simulink model "DVBS2BentPipeLinkModel"  (R2021b)
settings: Solver=VariableStepAuto  StartTime=0.0  StopTime=0.025  RelTol=1e-3
PreLoadFcn:
  | modulationAndCodingMode = 'QPSK 1/4';
  | seed = 25;
  | ldpcFrameLength = 'Normal';
  | selDPD = false;
  | ulFreq = 4;  % GHz
  | selLvlBO = 1;  % '30 dB  (negligible nonlinearity)'
  | gsTxAntDiam = 4;  % m
  | selDoppler = 1;  %'0 Hz'
  | filterSpanInSymbols = 6;
  | sampPerSym = 8;
  | altitude = 35600;  % km
  | satRxAntDiam = 0.3;  % m
  | satRxNoiseFigure = 6;  % dB
  | chebyFilterOrder = 4;
  | satHPABackoff = 8;  % dB
  | dlFreq = 4.2;  % GHz
  | satTxAntDiam = 0.3;  % m
  | gsRxAntDiam = 1;  % m
  | gsRxNoiseFigure = 3;  % dB
  | selPhNo = 1;  % 'Negligible (-100 dBc/Hz @ 100 Hz)'
  | iqAmpImbal = 0;  % dB
  | iqPhImbal = 0;  % deg
  | dcOffsetPct = 0;  % percent of mean in-phase voltage
  | selDcOffset = false;
  | selCorrIQ = false;
  | selCorrDoppler = false;
  | LDPCNumIterations = 50;
  | DVBS2BentPipeInit(modulationAndCodingMode, seed, ...
  |   ldpcFrameLength, selDPD, ...
  |   ulFreq, selLvlBO, gsTxAntDiam, selDoppler, ...
  |   filterSpanInSymbols, sampPerSym, ...
  |   altitude, satRxAntDiam, satRxNoiseFigure, ...
  |   chebyFilterOrder, satHPABackoff, dlFreq, satTxAntDiam, ...
  |   gsRxAntDiam, gsRxNoiseFigure, selPhNo, ...
  |   iqAmpImbal, iqPhImbal, dcOffsetPct, ...
  |   selDcOffset, selCorrIQ, selCorrDoppler, ...
  |   LDPCNumIterations);
  | 
  | clear modulationAndCodingMode seed ldpcFrameLength selDPD
  | clear ulFreq selLvlBO gsTxAntDiam selDoppler
  | clear filterSpanInSymbols sampPerSym
  | clear altitude satRxAntDiam satRxNoiseFigure
  | clear chebyFilterOrder satHPABackoff dlFreq satTxAntDiam
  | clear gsRxAntDiam gsRxNoiseFigure selPhNo
  | clear iqAmpImbal iqPhImbal dcOffsetPct
  | clear selDcOffset selCorrIQ selCorrDoppler
  | clear LDPCNumIterations
undefined symbols (not defined in the file or in its folder): paramRFSatLink
libraries: dspstat3 x17, commrflib2 x9, commrfcorlib x5, commblkcod2 x4, dspsigops x4, commsink2 x3, commutil2 x3, dspmathops x3, commblkintrlv2 x2, dspobslib x2, commdigbbndpm3 x2, commfilt2 x2
(part 1 of 2)
settings Model: Creator=The MathWorks, Inc.  LastModifiedBy=lenovo

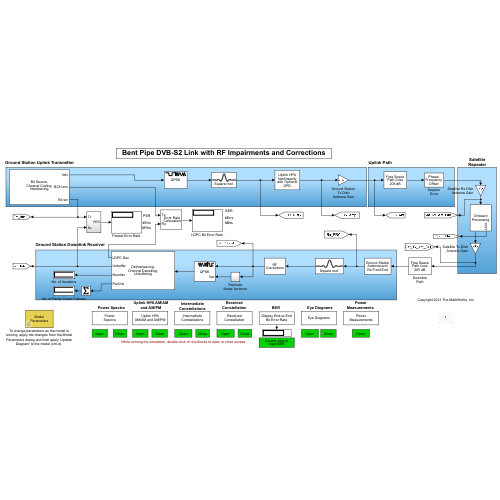
[thumbnail: Simulink's stored preview of the top-level diagram]
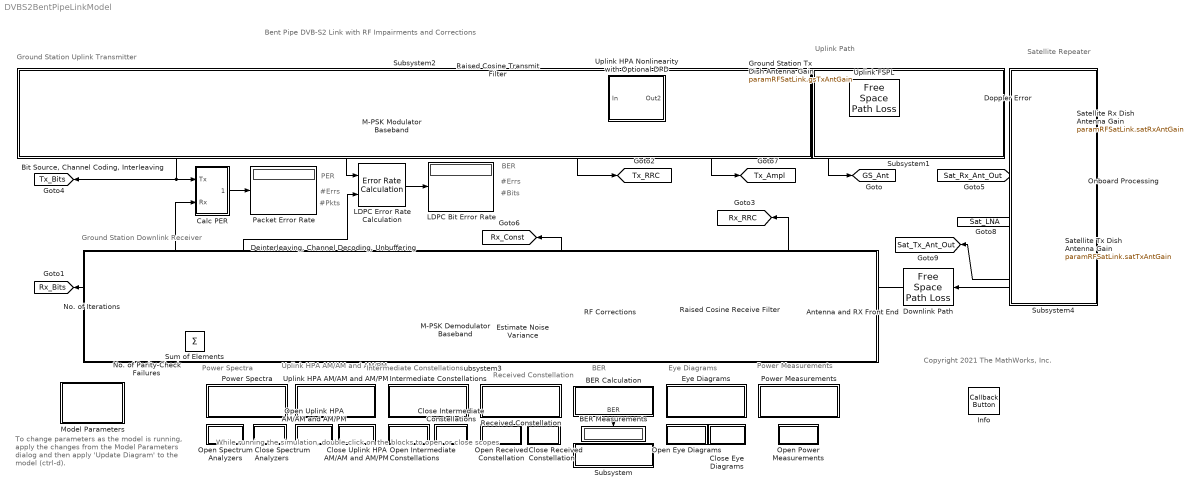
== system DVBS2BentPipeLinkModel ==
  note: Copyright 2021 The MathWorks, Inc.
  note: BER
  note: PER
  note: Satellite
      | Repeater
  note: Ground Station Uplink Transmitter
  note: To change parameters as the model is running, apply the changes from the Model Parameters dialog and then apply 'Update Diagram' to the model (ctrl-d).
  note: Received
      | Constellation
  note: Eye Diagrams
  note: BER
  note: While running the simulation, double-click on the blocks to open or close scopes
  note: Uplink HPA AM/AM
      | and AM/PM
  note: #Pkts
  note: #Errs
  note: Ground Station Downlink Receiver
  note: Bent Pipe DVB-S2 Link with RF Impairments and Corrections
  note: #Bits
  note: #Errs
  note: Power Spectra
  note: Intermediate
      | Constellations
  note: Uplink Path
  note: Power
      | Measurements
  Antenna and RX Front End : Subsystem
      mask Display: disp('Ground Station\nAntenna and\nRx Front End')
  BER Calculation : Subsystem
      mask Display: disp('Display End-to-End\nBit Error Rate');
  BER Measurements : Display
      settings: Format=short_e
  "Bit Source, Channel Coding, Interleaving" : Subsystem
      mask Display:
      | disp('Bit Source,\nChannel Coding,\nInterleaving\n')
      | port_label('output',1,'Intlv')
      | port_label('output',2,'BCH enc')
      | port_label('output',3,'Bit src')
  Calc PER : Subsystem
  Close Intermediate Constellations : Subsystem
      settings: OpenFcn=|
      | % RRC signal before and after uplink HPA
      | ULHPACD = [bdroot '/Intermediate Constellations/RRC Signal Before and After Uplink HPA'];
      | close_system(ULHPACD);
      | % set_param(ULHPACD,'OpenScopeAtSimStart','off');
      | clear ULHPACD
      | 
      | % Constellations onboard satellite
      | onboardCD = [bdroot '/Intermediate Constellations/Onboard Constellations'];
      | close_system(onboardCD);
      | % set_param(onboardCD,'OpenScopeAtSimStart','off');
      | clear onboardCD
      mask Display: disp('Close');
  Close Eye Diagrams : Subsystem
      settings: OpenFcn=|
      | % Satellite AGC Output Eye Diagram
      | satAGCED = [bdroot '/Eye Diagrams/Sat AGC Output Eye Diagram'];
      | close_system(satAGCED);
      | % set_param(satAGCED,'OpenScopeAtSimStart','off');
      | clear satAGCED
      | 
      | % Chebyshev Filter Output Eye Diagram
      | chebyFiltED = [bdroot '/Eye Diagrams/Chebyshev Filter Output Eye Diagram'];
      | close_system(chebyFiltED);
      | % set_param(chebyFiltED,'OpenScopeAtSimStart','off');
      | clear chebyFiltED
      | 
      | % Rx Eye Diagram
      | rxED = [bdroot '/Eye Diagrams/Rx Eye Diagram'];
      | close_system(rxED);
      | % set_param(rxED,'OpenScopeAtSimStart','off');
      | clear rxED
      mask Display: disp('Close');
  Close Received Constellation : Subsystem
      settings: OpenFcn=|
      | rxCD = [bdroot '/Received Constellation/Received Constellation'];
      | close_system(rxCD);
      | % set_param(rxCD,'OpenScopeAtSimStart','off');
      | clear rxCD
      mask Display: disp('Close');
  Close Spectrum Analyzers : Subsystem
      settings: OpenFcn=|
      | % Tx and rx spectra
      | txrxSA = [bdroot '/Power Spectra/Ground Station Tx and Rx Spectra'];
      | close_system(txrxSA);
      | % set_param(txrxSA,'OpenScopeAtSimStart','off');
      | clear txrxSA
      | 
      | % Spectra onboard satellite
      | satSA = [bdroot '/Power Spectra/Onboard Spectra'];
      | close_system(satSA);
      | % set_param(satSA,'OpenScopeAtSimStart','off');
      | clear satSA
      mask Display: disp('Close');
  Close Uplink HPA AM/AM and AM/PM : Subsystem
      settings: OpenFcn=|
      | % AM/AM
      | AMAMplot = [bdroot '/Uplink HPA AM//AM and AM//PM/Input&Output of HPA/HPA AM to AM'];
      | close_system(AMAMplot);
      | % set_param(AMAMplot,'OpenScopeAtSimStart','off');
      | clear AMAMplot
      | 
      | % AM/PM
      | AMPMplot = [bdroot '/Uplink HPA AM//AM and AM//PM/Input&Output of HPA/HPA AM to PM'];
      | close_system(AMPMplot);
      | % set_param(AMPMplot,'OpenScopeAtSimStart','off');
      | clear AMPMplot
      mask Display: disp('Close');
  "Deinterleaving, Channel Decoding, Unbuffering" : Subsystem
      mask Display:
      | disp('Deinterleaving,\nChannel Decoding,\nUnbuffering')
      | port_label('output',1,'LDPC Dec')
      | port_label('output',2,'Unbuffer')
      | port_label('output',3,'NumIter')
      | port_label('output',4,'ParChk')
  Doppler Error : commrflib2/Phase// Frequency Offset  phaseOffset=0  freqPort=off  freqOffset=paramRFSatLink.DoppOffset
  Downlink Path : commrflib2/Free Space Path Loss  mode=Distance and Frequency  dB=180  d=paramRFSatLink.Altitude  fc="paramRFSatLink.DownlinkFrequency * 1e3  % GHz to MHz"
      settings: SourceProductBaseCode=CM
  Estimate Noise Variance : Subsystem
  Eye Diagrams : Subsystem
      mask Display: disp('Eye Diagrams');
  Ground Station Tx Dish Antenna Gain : Gain  Gain=paramRFSatLink.gsTxAntGain  SaturateOnIntegerOverflow=on  OutDataTypeStr=Inherit: Same as input  ParamDataTypeStr=Inherit: Same as input
  Info : CallbackButton  ButtonText=?
      settings: ClickFcn=showExample('satcom/DVBS2BentPipeSimulationWithRFImpairmentsAndCorrectionsExample')
  Intermediate Constellations : Subsystem
      mask Display: disp('Intermediate\nConstellations')
  LDPC Bit Error Rate : Display
  LDPC Error Rate Calculation : commsink2/Error Rate Calculation  N=paramRFSatLink.LDPCLinkRecDelay  st_delay=paramRFSatLink.BCHCodewordLength  cp_mode=Entire frame  subframe=[]  PMode=Port  WsName=ErrorVec  RsMode2=off  stop=off  numErr=100  maxBits=1e6
  M-PSK Demodulator Baseband : commdigbbndpm3/M-PSK Demodulator Baseband  M=paramRFSatLink.ModulationOrder  OutType=Bit  DecType=Approximate log-likelihood ratio  VarSource=Port  Variance=1/(1+10^(paramRFSatLink.EsNodB/10))  Dec=User-defined  Mapping=paramRFSatLink.SymbolMapping  Ph=paramRFSatLink.PhaseOffset  outDtype1=double  outDtype2=double  derotateFactorWordLen=16  derotateFactorDataTypeStr=Inherit: Same word length as input  derotateFactorLastDataTypeStr=Inherit: Same word length as input
  M-PSK Modulator Baseband : commdigbbndpm3/M-PSK Modulator Baseband  M=paramRFSatLink.ModulationOrder  InType=Bit  Enc=User-defined  Mapping=paramRFSatLink.SymbolMapping  Ph=paramRFSatLink.PhaseOffset  outDtype=double  outWordLen=16  outUDDataType=sfix(16)  outFracLenMode=Best precision  outFracLen=15  outDataTypeStr=double  outLastDataTypeStr=double
  Model Parameters : Subsystem  mask(Model Parameters){modulationAndCodingMode=QPSK 1/4, seed=23, ldpcFrameLength=Normal, selDPD=off, ulFreq=14, selLvlBO=30 dB  (negligible nonlinearity), gsTxAntDiam=8, dopplerFreq=0, filterSpanInSymbols=6, sampPerSym=8, altitude=35600, satRxAntDiam=2, satRxNoiseFigure=6, chebyFilterOrder=4, satHPABackoff=4, dlFreq=12, satTxAntDiam=2, gsRxAntDiam=8, gsRxNoiseFigure=3, selPhNo=Negligible (-100 dBc/Hz @ 100 Hz), iqAmpImbal=0, iqPhImbal=0, dcOffsetPct=0, selCorrDCOffset=off, selCorrIQ=off, selCorrDoppler=off, LDPCNumIterations=50}
      mask prompts: modulationAndCodingMode "Mode:"; seed "Seed (for random data and noise):"; ldpcFrameLength "LDPC frame length:"; selDPD "Digital predistortion"; ulFreq "Uplink frequency (GHz):"; selLvlBO "HPA backoff level:"; gsTxAntDiam "Transmit antenna diameter (m):"; dopplerFreq "Doppler error (Hz):"; filterSpanInSymbols "Filter span (symbols):"; sampPerSym "Filter output samples per symbol:"; altitude "Satellite altitude (km):"; satRxAntDiam "Receive antenna diameter (m):"; satRxNoiseFigure "Receiver noise figure (dB):"; chebyFilterOrder "Chebyshev filter order:"; satHPABackoff "HPA backoff level (dB):"; dlFreq "Downlink frequency (GHz):"; satTxAntDiam "Transmit antenna diameter (m):"; gsRxAntDiam "Receive antenna diameter (m):"; gsRxNoiseFigure "Receiver noise figure (dB):"; selPhNo "Phase noise:"; iqAmpImbal "I/Q amplitude imbalance (dB):"; iqPhImbal "I/Q phase imbalance (deg):"; dcOffsetPct "In-phase DC offset (%):"; selCorrDCOffset "DC offset correction"; selCorrIQ "I/Q imbalance correction"; selCorrDoppler "Doppler correction"; LDPCNumIterations "Number of LDPC decoder iterations:"
      mask help:
      | Select the scenarios from the mask to change the link parameters. Each of the mask parameters sets the parameters in the corresponding RF impairment or corresponding correction block(s).
      |
      | To make changes as the model is running, apply the changes from this dialog and then apply Update Diagram to the model (crtl-d).
      mask init:
      | DVBS2BentPipeInit(modulationAndCodingMode, seed, ...
      |   ldpcFrameLength, selDPD, ulFreq, selLvlBO, ...
      |   gsTxAntDiam, dopplerFreq, filterSpanInSymbols, ...
      |   sampPerSym, altitude, satRxAntDiam, satRxNoiseFigure, ...
      |   chebyFilterOrder, satHPABackoff, dlFreq, satTxAntDiam, ...
      |   gsRxAntDiam, gsRxNoiseFigure, selPhNo, ...
      |   iqAmpImbal, iqPhImbal, dcOffsetPct, ...
      |   selCorrDCOffset, selCorrIQ, selCorrDoppler, ...
      |   LDPCNumIterations);
      mask Help: helpview(commdhelp);
      mask TypeOptions modulationAndCodingMode: QPSK 1/4 | QPSK 1/3 | QPSK 2/5 | QPSK 1/2 | QPSK 3/5 | QPSK 2/3 | QPSK 3/4 | QPSK 4/5 | QPSK 5/6 | QPSK 8/9 | QPSK 9/10 | 8PSK 3/5 | 8PSK 2/3 | 8PSK 3/4 | 8PSK 5/6 | 8PSK 8/9 | 8PSK 9/10
      mask TypeOptions ldpcFrameLength: Normal | Short
      mask TypeOptions selLvlBO: 30 dB  (negligible nonlinearity) | 7 dB  (moderate nonlinearity) | 1 dB  (severe nonlinearity)
      mask TypeOptions selPhNo: Negligible (-100 dBc/Hz @ 100 Hz) | Low  (-55 dBc/Hz @ 100 Hz) | High  (-48 dBc/Hz @ 100 Hz)
      mask DialogControl uplinkTab Prompt: Uplink
      mask DialogControl satelliteTab Prompt: Satellite
      mask DialogControl downlinkTab Prompt: Downlink
      mask Display: disp('Model\nParameters');
  No. of Iterations : Display
  No. of Parity-Check Failures : Display
  Onboard Processing : Subsystem
      mask Display:
      | disp('Onboard\nProcessing');
      | port_label('output',2,'LNA');
  Open Intermediate Constellations : Subsystem
      settings: OpenFcn=|
      | % RRC signal before and after uplink HPA
      | ULHPACD = [bdroot '/Intermediate Constellations/RRC Signal Before and After Uplink HPA'];
      | open_system(ULHPACD);
      | % set_param(ULHPACD,'OpenScopeAtSimStart','on');
      | clear ULHPACD
      | 
      | % Constellations onboard satellite
      | onboardCD = [bdroot '/Intermediate Constellations/Onboard Constellations'];
      | open_system(onboardCD);
      | % set_param(onboardCD,'OpenScopeAtSimStart','on');
      | clear onboardCD
      mask Display: disp('Open');
  Open Eye Diagrams : Subsystem
      settings: OpenFcn=|
      | % Satellite AGC Output Eye Diagram
      | satAGCED = [bdroot '/Eye Diagrams/Sat AGC Output Eye Diagram'];
      | open_system(satAGCED);
      | % set_param(satAGCED,'OpenScopeAtSimStart','on');
      | clear satAGCED
      | 
      | % Chebyshev Filter Output Eye Diagram
      | chebyFiltED = [bdroot '/Eye Diagrams/Chebyshev Filter Output Eye Diagram'];
      | open_system(chebyFiltED);
      | % set_param(chebyFiltED,'OpenScopeAtSimStart','on');
      | clear chebyFiltED
      | 
      | % Rx Eye Diagram
      | rxED = [bdroot '/Eye Diagrams/Rx Eye Diagram'];
      | open_system(rxED);
      | % set_param(rxED,'OpenScopeAtSimStart','on');
      | clear rxED
      mask Display: disp('Open');
  Open Power Measurements : Subsystem
      settings: OpenFcn=open_system([bdroot '/Power Measurements']);
      mask Display: disp('Open');
  Open Received Constellation : Subsystem
      settings: OpenFcn=|
      | rxCD = [bdroot '/Received Constellation/Received Constellation'];
      | open_system(rxCD);
      | % set_param(rxCD,'OpenScopeAtSimStart','on');
      | clear rxCD
      mask Display: disp('Open');
  Open Spectrum Analyzers : Subsystem
      settings: OpenFcn=|
      | % Tx and rx spectra
      | txrxSA = [bdroot '/Power Spectra/Ground Station Tx and Rx Spectra'];
      | open_system(txrxSA);
      | % set_param(txrxSA,'OpenScopeAtSimStart','on');
      | clear txrxSA
      | 
      | % Spectra onboard satellite
      | satSA = [bdroot '/Power Spectra/Onboard Spectra'];
      | open_system(satSA);
      | % set_param(satSA,'OpenScopeAtSimStart','on');
      | clear satSA
      mask Display: disp('Open');
  Open Uplink HPA AM/AM and AM/PM : Subsystem
      settings: OpenFcn=|
      | % AM/AM
      | AMAMplot = [bdroot '/Uplink HPA AM//AM and AM//PM/Input&Output of HPA/HPA AM to AM'];
      | open_system(AMAMplot);
      | % set_param(AMAMplot,'OpenScopeAtSimStart','on');
      | clear AMAMplot
      | 
      | % AM/PM
      | AMPMplot = [bdroot '/Uplink HPA AM//AM and AM//PM/Input&Output of HPA/HPA AM to PM'];
      | open_system(AMPMplot);
      | % set_param(AMPMplot,'OpenScopeAtSimStart','on');
      | clear AMPMplot
      mask Display: disp('Open');
  Packet Error Rate : Display
  Power Measurements : Subsystem
      mask Display: disp('Power\nMeasurements')
  Power Spectra : Subsystem
      mask Display: disp('Power\nSpectra')
  RF Corrections : Subsystem
      mask Display: disp('RF\nCorrections')
  Raised Cosine Receive Filter : commfilt2/Raised Cosine Receive Filter  filtType=Square root  R=0.25  filtSpan=paramRFSatLink.FilterSpanInSymbols  N=paramRFSatLink.SamplesPerSymbol  downFactor=paramRFSatLink.SamplesPerSymbol  downOffset=0  filterGain=1/sqrt(paramRFSatLink.SamplesPerSymbol)  InputProcessing=Columns as channels (frame based)  RateOptions=Enforce single-rate processing  framing=Mute  checkCoeff=off  variableName=rcRxFilt  currentFiltSpan=paramRFSatLink.FilterSpan  D=(paramRFSatLink.FilterSpan)/2  inputOffset=0  sampMode=Mute  saveAsFlag=0  rateMode=Downsampling  checkGain=Normalized  launchFVT=off  roundingMode=Floor  overflowMode=off  coeffDataTypeStr=Inherit: Same word length as input  coeffMin=[]  coeffMax=[]  coeffLastDataTypeStr=Inherit: Same word length as input  accumDataTypeStr=Inherit: Same as product output  accumLastDataTypeStr=Inherit: Same as product output  outputDataTypeStr=Inherit: Same as accumulator  outputMin=[]  outputMax=[]  outputLastDataTypeStr=Inherit: Same as accumulator
  Raised Cosine Transmit Filter : commfilt2/Raised Cosine Transmit Filter  filtType=Square root  R=0.25  filtSpan=paramRFSatLink.FilterSpanInSymbols  N=paramRFSatLink.SamplesPerSymbol  filterGain=sqrt(paramRFSatLink.SamplesPerSymbol)  InputProcessing=Columns as channels (frame based)  RateOptions=Enforce single-rate processing  framing=Mute  checkCoeff=off  variableName=rcTxFilt  checkGain=Normalized  sampMode=Mute  saveAsFlag=0  currentFiltSpan=paramRFSatLink.FilterSpan  D=(paramRFSatLink.FilterSpan)/2  launchFVT=off  roundingMode=Floor  overflowMode=off  coeffDataTypeStr=Inherit: Same word length as input  coeffMin=[]  coeffMax=[]  coeffLastDataTypeStr=Inherit: Same word length as input  outputDataTypeStr=Inherit: Same as accumulator  outputMin=[]  outputMax=[]  outputLastDataTypeStr=Inherit: Same as accumulator
  Received Constellation : Subsystem
      mask Display: disp('Received\nConstellation')
  Satellite Rx Dish Antenna Gain : Gain  Gain=paramRFSatLink.satRxAntGain  SaturateOnIntegerOverflow=on  OutDataTypeStr=Inherit: Same as input  ParamDataTypeStr=Inherit: Same as input
  Satellite Tx Dish Antenna Gain : Gain  Gain=paramRFSatLink.satTxAntGain  SaturateOnIntegerOverflow=on  OutDataTypeStr=Inherit: Same as input  ParamDataTypeStr=Inherit: Same as input
  Subsystem : Subsystem
      settings: OpenFcn=|
      | % Set value to reset BER
      | warning('off', 'Simulink:Engine:NonTunableVarChanged');
      | paramRFSatLink.resetBER = 1;
      | set_param(bdroot, 'SimulationCommand', 'update');
      | pause(0.1)
      | 
      | % Set value so that BER is not continually reset
      | paramRFSatLink.resetBER = 0;
      | set_param(bdroot, 'SimulationCommand', 'update');
      | warning('on', 'Simulink:Engine:NonTunableVarChanged');
      mask Display: disp('Double-click to\nreset BER')
  Subsystem1 : Subsystem
  Subsystem2 : Subsystem
  Subsystem3 : Subsystem
  Subsystem4 : Subsystem
  Sum of Elements : Sum  Inputs=+
  Uplink FSPL : commrflib2/Free Space Path Loss  mode=Distance and Frequency  dB=180  d=paramRFSatLink.Altitude  fc="paramRFSatLink.UplinkFrequency * 1e3  % GHz to MHz"
      settings: SourceProductBaseCode=CM
  Uplink HPA Nonlinearity with Optional DPD : Subsystem
      mask Display: disp('Uplink HPA\nNonlinearity\nwith Optional\nDPD')
  Uplink HPA AM/AM and AM/PM : Subsystem
      mask Display: disp('Uplink HPA\nAM/AM and AM/PM')
  tag scope: GS_Ant=global, Rx_Bits=global, Rx_Const=global, Rx_RRC=global, Sat_LNA=global, Sat_Rx_Ant_Out=global, Sat_Tx_Ant_Out=global, Tx_Ampl=global, Tx_Bits=global, Tx_RRC=global
  wires:
  Satellite Rx Dish Antenna Gain/1 -> Onboard Processing/1(In1), [Sat_Rx_Ant_Out]
  LDPC Error Rate Calculation/1 -> LDPC Bit Error Rate/1
  Raised Cosine Transmit Filter/1 -> Uplink HPA Nonlinearity with Optional DPD/1(In), [Tx_RRC]
  Sum of Elements/1 -> No. of Parity-Check Failures/1
  Antenna and RX Front End/1(Out1) -> Raised Cosine Receive Filter/1, [Rx_RRC]
  Doppler Error/1 -> Satellite Rx Dish Antenna Gain/1
  BER Calculation/1(BER) -> BER Measurements/1
  Satellite Tx Dish Antenna Gain/1 -> [Sat_Tx_Ant_Out], Downlink Path/1
  Estimate Noise Variance/1(Out1) -> M-PSK Demodulator Baseband/2
  Calc PER/1(PER) -> Packet Error Rate/1
  Uplink HPA Nonlinearity with Optional DPD/1(Out2) -> Ground Station Tx Dish Antenna Gain/1, [Tx_Ampl]
  Downlink Path/1 -> Antenna and RX Front End/1(In1)
  Uplink FSPL/1 -> Doppler Error/1
  Ground Station Tx Dish Antenna Gain/1 -> [GS_Ant], Uplink FSPL/1
  "Bit Source, Channel Coding, Interleaving"/3(Bit Src) -> [Tx_Bits], Calc PER/1(Tx)
  "Bit Source, Channel Coding, Interleaving"/1(Intlv Out) -> M-PSK Modulator Baseband/1
  "Bit Source, Channel Coding, Interleaving"/2(BCH Enc Out) -> LDPC Error Rate Calculation/1
  "Deinterleaving, Channel Decoding, Unbuffering"/2(Unbuffer) -> [Rx_Bits], Calc PER/2(Rx)
  M-PSK Demodulator Baseband/1 -> "Deinterleaving, Channel Decoding, Unbuffering"/1(QPSK Demod)
  "Deinterleaving, Channel Decoding, Unbuffering"/1(LDPC Dec) -> LDPC Error Rate Calculation/2
  "Deinterleaving, Channel Decoding, Unbuffering"/3(NumIter) -> No. of Iterations/1
  "Deinterleaving, Channel Decoding, Unbuffering"/4(ParChk) -> Sum of Elements/1
  Onboard Processing/1(Out2) -> Satellite Tx Dish Antenna Gain/1
  Onboard Processing/2(LNA Out) -> [Sat_LNA]
  Raised Cosine Receive Filter/1 -> RF Corrections/1(In1)
  M-PSK Modulator Baseband/1 -> Raised Cosine Transmit Filter/1
  RF Corrections/1(Out1) -> Estimate Noise Variance/1(In1), M-PSK Demodulator Baseband/1, [Rx_Const]

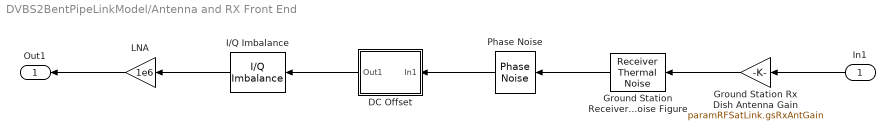
== system DVBS2BentPipeLinkModel/Antenna and RX Front End ==
  In1 : Inport
  DC Offset : Subsystem
      mask Display: disp('DC Offset')
  Ground Station Receiver Noise Figure : commrflib2/Receiver Thermal Noise  method=Noise figure  ntemp=paramRFSatLink.RXTemp  nfigure=paramRFSatLink.GSRxNoiseFigure  nfactor=2  add290KAntennaNoise=off  seed=67987
      settings: SourceProductBaseCode=CM
  Ground Station Rx Dish Antenna Gain : Gain  Gain=paramRFSatLink.gsRxAntGain  SaturateOnIntegerOverflow=on  OutDataTypeStr=Inherit: Same as input  ParamDataTypeStr=Inherit: Same as input
  I/Q Imbalance : commrflib2/I//Q Imbalance  ampImbal=paramRFSatLink.IQAmpImbal  phsImbal=paramRFSatLink.IQPhImbal  Idc=0  Qdc=0
      settings: SourceProductBaseCode=CM
  LNA : Gain  Gain=1e6
  Phase Noise : impairlib/Phase Noise  Level=paramRFSatLink.PhaseNoise  FrequencyOffset=100  SampleRate=2e5  RandomStream=mt19937ar with seed  Seed=2137  SimulateUsing=Interpreted execution
      settings: SourceProductBaseCode=CM,AM,SX
  Out1 : Outport  VectorParamsAs1DForOutWhenUnconnected=off
  wires:
  LNA/1 -> Out1/1
  Ground Station Receiver Noise Figure/1 -> Phase Noise/1
  In1/1 -> Ground Station Rx Dish Antenna Gain/1
  I/Q Imbalance/1 -> LNA/1
  Ground Station Rx Dish Antenna Gain/1 -> Ground Station Receiver Noise Figure/1
  DC Offset/1(Out1) -> I/Q Imbalance/1
  Phase Noise/1 -> DC Offset/1(In1)

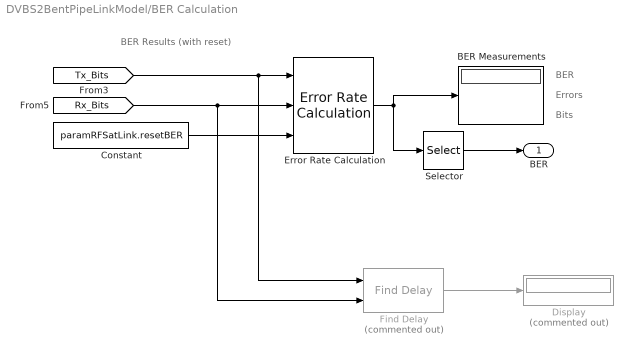
== system DVBS2BentPipeLinkModel/BER Calculation ==
  note: BER
  note: Errors
  note: Bits
  note: BER Results (with reset)
  BER Measurements : Display
  Constant : Constant  Value=paramRFSatLink.resetBER  SampleTime=Inf
  Display : Display  Commented=on
  Error Rate Calculation : commsink2/Error Rate Calculation  N=paramRFSatLink.FullLinkRecDelay  st_delay=paramRFSatLink.BCHMessageLength  cp_mode=Entire frame  subframe=[]  PMode=Port  WsName=ErrorVec  RsMode2=on  stop=off  numErr=200  maxBits=1e6
  Find Delay : commutil2/Find Delay  Commented=on  corrLength=15000  chgSigOP=off  stopUpdate=off  numConstDelay=3
      settings: SourceProductBaseCode=CM
  Selector : Selector  InputPortWidth=3  IndexOptions=Index vector (dialog)  Indices=[1]  OutputSizes=1
  BER : Outport  VectorParamsAs1DForOutWhenUnconnected=off
  wires:
  [Rx_Bits] -> Find Delay/2, Error Rate Calculation/2
  Error Rate Calculation/1 -> Selector/1, BER Measurements/1
  Constant/1 -> Error Rate Calculation/3
  Selector/1 -> BER/1
  [Tx_Bits] -> Find Delay/1, Error Rate Calculation/1
  Find Delay/1 -> Display/1

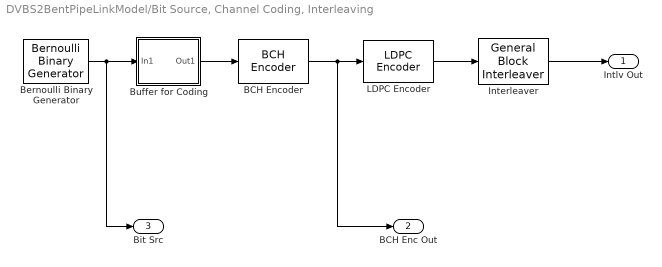
== system DVBS2BentPipeLinkModel/Bit Source, Channel Coding, Interleaving ==
  BCH Encoder : commblkcod2/BCH Encoder  n=paramRFSatLink.BCHCodewordLength  k=paramRFSatLink.BCHMessageLength  specShortening=off  shortenedK=5  specGenPoly=on  genPoly=paramRFSatLink.BCHGeneratorPoly  specPrimPoly=on  prPoly=paramRFSatLink.BCHPrimitivePoly  specDisableGenCheck=on  specPuncture=off  punctVec=[ones(8,1); zeros(2,1)]
      settings: SourceProductBaseCode=CM
  Bernoulli Binary Generator : commrandsrc3/Bernoulli Binary Generator  ProbabilityOfZero=0.5  SeedSource=Parameter  Seed=paramRFSatLink.Seed  SampleTime=paramRFSatLink.BitPeriod  SamplesPerFrame=paramRFSatLink.NumBitsPerPacket  OutputDataType=double  SimulateUsing=Interpreted execution
  Buffer for Coding : Subsystem
      mask Display: disp('BBFRAME\nBuffering')
  Interleaver : commblkintrlv2/General Block Interleaver  permutationVectorSource=Dialog  elements=paramRFSatLink.InterleaveOrder
      settings: SourceProductBaseCode=CM
  LDPC Encoder : commblkcod2/LDPC Encoder  ParityCheckMat=paramRFSatLink.LDPCParityCheckMatrix
      settings: SourceProductBaseCode=CM
  Intlv Out : Outport
  BCH Enc Out : Outport  Port=2
  Bit Src : Outport  Port=3
  wires:
  Bernoulli Binary Generator/1 -> Bit Src/1, Buffer for Coding/1(In1)
  Buffer for Coding/1(Out1) -> BCH Encoder/1
  Interleaver/1 -> Intlv Out/1
  BCH Encoder/1 -> BCH Enc Out/1, LDPC Encoder/1
  LDPC Encoder/1 -> Interleaver/1

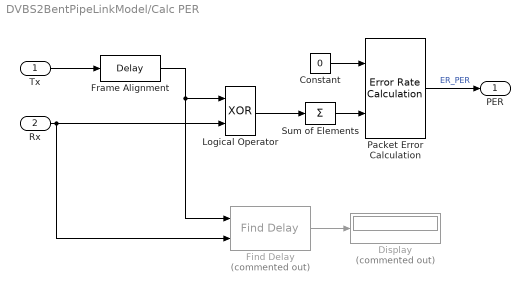
== system DVBS2BentPipeLinkModel/Calc PER ==
  Tx : Inport
  Rx : Inport  Port=2
  Constant : Constant  Value=0  OutDataTypeStr=double
  Display : Display  Commented=on
  Find Delay : commutil2/Find Delay  Commented=on  corrLength=6000  chgSigOP=off  stopUpdate=off  numConstDelay=3
      settings: SourceProductBaseCode=CM
  Frame Alignment : dspobslib/Delay  InputProcessing=Columns as channels (frame based)  dly_unit=Samples  delay=paramRFSatLink.FullLinkRecDelay  ic_detail=off  dif_ic_for_ch=off  dif_ic_for_dly=off  ic=0  reset_popup=None
      settings: SourceProductBaseCode=DS
  Logical Operator : Logic  Operator=XOR  AllPortsSameDT=off  OutDataTypeStr=boolean
  Packet Error Calculation : commsink2/Error Rate Calculation  N=0  st_delay=2*paramRFSatLink.NumInfoBitsPerCodeword/paramRFSatLink.NumBitsPerPacket  cp_mode=Entire frame  subframe=[]  PMode=Port  WsName=ErrorVec  RsMode2=off  stop=off  numErr=100  maxBits=1e6
  Sum of Elements : Sum  Inputs=+  OutDataTypeStr=double
  PER : Outport  VectorParamsAs1DForOutWhenUnconnected=off
  wires:
  Constant/1 -> Packet Error Calculation/1
  Rx/1 -> Find Delay/2, Logical Operator/2
  Packet Error Calculation/1 -> PER/1  "ER_PER"
  Tx/1 -> Frame Alignment/1
  Frame Alignment/1 -> Find Delay/1, Logical Operator/1
  Logical Operator/1 -> Sum of Elements/1
  Sum of Elements/1 -> Packet Error Calculation/2
  Find Delay/1 -> Display/1

== system DVBS2BentPipeLinkModel/Close Intermediate Constellations ==

== system DVBS2BentPipeLinkModel/Close Eye Diagrams ==

== system DVBS2BentPipeLinkModel/Close Received Constellation ==

== system DVBS2BentPipeLinkModel/Close Spectrum Analyzers ==

== system DVBS2BentPipeLinkModel/Close Uplink HPA AM//AM and AM//PM ==

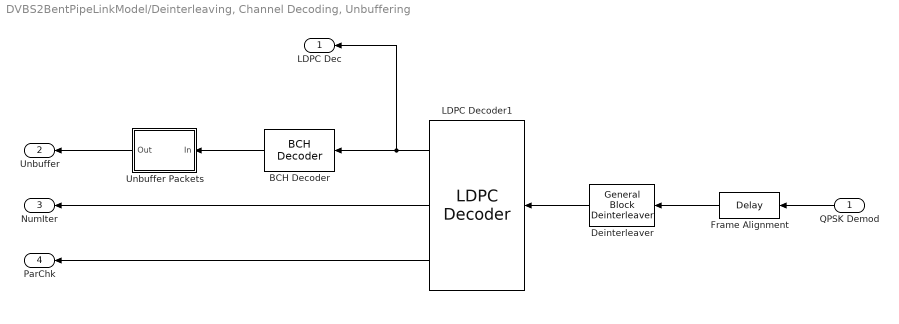
== system DVBS2BentPipeLinkModel/Deinterleaving, Channel Decoding, Unbuffering ==
  QPSK Demod : Inport
  BCH Decoder : commblkcod2/BCH Decoder  n=paramRFSatLink.BCHCodewordLength  k=paramRFSatLink.BCHMessageLength  specShortening=off  shortenedK=5  specGenPoly=on  genPoly=paramRFSatLink.BCHGeneratorPoly  specPrimPoly=on  prPoly=paramRFSatLink.BCHPrimitivePoly  specDisableGenCheck=on  specPuncture=off  punctVec=[ones(8,1); zeros(2,1)]  specErasurePort=off  showNumErr=off
      settings: SourceProductBaseCode=CM
  Deinterleaver : commblkintrlv2/General Block Deinterleaver  permutationVectorSource=Dialog  elements=paramRFSatLink.InterleaveOrder
      settings: SourceProductBaseCode=CM
  Frame Alignment : dspobslib/Delay  InputProcessing=Columns as channels (frame based)  dly_unit=Samples  delay=paramRFSatLink.RxFilterDelay  ic_detail=off  dif_ic_for_ch=off  dif_ic_for_dly=off  ic=0  reset_popup=None
      settings: SourceProductBaseCode=DS
  LDPC Decoder1 : commblkcod2/LDPC Decoder  ParityCheckMat=paramRFSatLink.LDPCParityCheckMatrix  OutputFmt=Information part  DecisionType=Hard decision  OutputDataType=double  NumIter=paramRFSatLink.LDPCNumIterations  DoParityCheck=on  OutputNumIter=on  OutputFinalChecks=on
      settings: SourceProductBaseCode=CM
  Unbuffer Packets : Subsystem
      mask Display: disp('BBFRAME\nUnbuffering')
  LDPC Dec : Outport
  Unbuffer : Outport  Port=2
  NumIter : Outport  Port=3
  ParChk : Outport  Port=4
  wires:
  Deinterleaver/1 -> LDPC Decoder1/1
  Unbuffer Packets/1(Out) -> Unbuffer/1
  LDPC Decoder1/2 -> NumIter/1
  Frame Alignment/1 -> Deinterleaver/1
  BCH Decoder/1 -> Unbuffer Packets/1(In)
  LDPC Decoder1/1 -> LDPC Dec/1, BCH Decoder/1
  QPSK Demod/1 -> Frame Alignment/1
  LDPC Decoder1/3 -> ParChk/1

== system DVBS2BentPipeLinkModel/Estimate Noise Variance ==
  In1 : Inport
  Constant : Constant  Value=paramRFSatLink.modIdx  SampleTime=-1
  Display : Display
  Estimate Noise Variance : MATLAB Function  TreatAsAtomicUnit=on
  Out1 : Outport  VectorParamsAs1DForOutWhenUnconnected=off
  wires:
  In1/1 -> Estimate Noise Variance/1(x)
  Constant/1 -> Estimate Noise Variance/2(modIdx)
  Estimate Noise Variance/1(estVar) -> Display/1, Out1/1

== system DVBS2BentPipeLinkModel/Eye Diagrams ==
  Chebyshev Filter Output Eye Diagram : EyeDiagram
  Rx Eye Diagram : EyeDiagram
  Sat AGC Output Eye Diagram : EyeDiagram
  wires:
  [Rx_RRC] -> Rx Eye Diagram/1
  [Sat_AGC_Out] -> Sat AGC Output Eye Diagram/1
  [Cheby_Filt_Out] -> Chebyshev Filter Output Eye Diagram/1

== system DVBS2BentPipeLinkModel/Intermediate Constellations ==
  Onboard Constellations : ConstellationDiagram  NumInputPorts=3
  RRC Signal Before and After Uplink HPA : ConstellationDiagram  NumInputPorts=2
  wires:
  [Tx_Ampl] -> RRC Signal Before and After Uplink HPA/2  "Uplink HPA Out"
  [Tx_RRC] -> RRC Signal Before and After Uplink HPA/1  "RRC Filter Out"
  [Sat_AGC_Out] -> Onboard Constellations/1  "LNA Out"
  [Cheby_Filt_Out] -> Onboard Constellations/2  "Chebyshev Filter Out"
  [Sat_PA_Out] -> Onboard Constellations/3  "PA Out"

== system DVBS2BentPipeLinkModel/Model Parameters ==

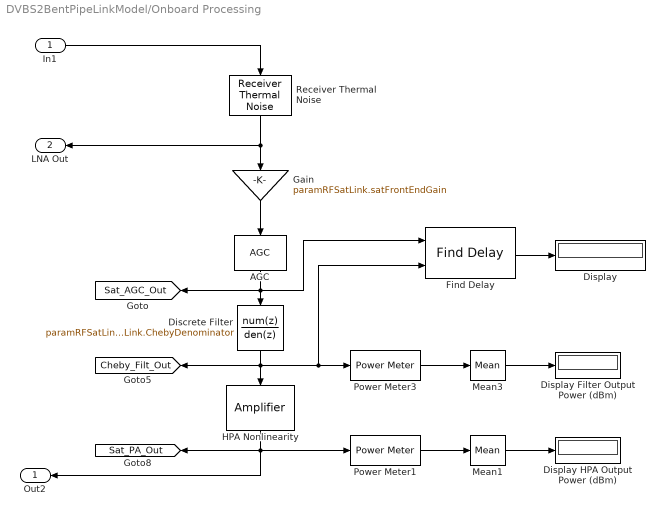
== system DVBS2BentPipeLinkModel/Onboard Processing ==
  In1 : Inport
  AGC : commrfcorlib/AGC  LegacyMode=off  DetectorMethod=Rectifier  LoopMethod=Linear  UpdatePeriod=100  StepSize=0.1  AdaptationStepSize=0.01  DesiredOutputPower=paramRFSatLink.AGCDesPout  AveragingLength=400  MaximumGain=30  MaxPowerGain=60  GainOutputPort=off  InputPowerOutputPort=off  SimulateUsing=Interpreted execution
  Discrete Filter : DiscreteFilter  Numerator=paramRFSatLink.ChebyNumerator  Denominator=paramRFSatLink.ChebyDenominator  InputProcessing=Columns as channels (frame based)
  Display : Display
  Display Filter Output Power (dBm) : Display
  Display HPA Output Power (dBm) : Display
  Find Delay : commutil2/Find Delay  corrLength=1000  chgSigOP=off  stopUpdate=off  numConstDelay=3
      settings: SourceProductBaseCode=CM
  Gain : Gain  Gain=paramRFSatLink.satFrontEndGain
  HPA Nonlinearity : commrflib2/Amplifier  Model=AM/AM - AM/PM  LinearGainDB=0  TOI_Type=IIP3  IIP3=Inf  OIP3=Inf  IP1dB=Inf  OP1dB=Inf  IPsat=Inf  OPsat=Inf  Table=paramRFSatLink.ampTable  MagnitudeGainDB=0  Vsat=1  MagnitudeSmooth=2  PhaseGainRadian=-.45  PhaseSaturation=.88  PhaseSmooth=3.43  InputScaleDB=0  AmAmParameters=[ 2.1587, 1.1517 ]  AmPmParameters=[ 4.0033, 9.1040 ]  OutputScaleDB=0  SimulateUsing=Code generation  IncludeNoise=off  NoiseType=Noise temperature  NoiseTemperature=290  NoiseFigure=10 * log10( 2 )  NoiseFactor=2  SeedSource=Auto  Seed=67987
      settings: SourceProductBaseCode=CM
  Mean1 : dspstat3/Mean  run=off  InputProcessing=Columns as channels (frame based)  reset_popup=None  directionMode=Each column  dimension=1  roiEnable=off  roiType=Rectangles  roiPortion=Entire ROI  roiOutput=Individual statistics for each ROI  roiFlag=off  roundingMode=Floor  overflowMode=off  outputDataTypeStr=Inherit: Same as accumulator  outputMin=[]  outputMax=[]  outputLastDataTypeStr=Inherit: Same as accumulator
  Mean3 : dspstat3/Mean  run=off  InputProcessing=Columns as channels (frame based)  reset_popup=None  directionMode=Each column  dimension=1  roiEnable=off  roiType=Rectangles  roiPortion=Entire ROI  roiOutput=Individual statistics for each ROI  roiFlag=off  roundingMode=Floor  overflowMode=off  outputDataTypeStr=Inherit: Same as accumulator  outputMin=[]  outputMax=[]  outputLastDataTypeStr=Inherit: Same as accumulator
  Power Meter1 : dspstat3/Power Meter  Measurement=Average power  WindowLength=2000  ReferenceLoad=1  PowerUnits=dBm  SimulateUsing=Code generation
      settings: SourceProductBaseCode=DS
  Power Meter3 : dspstat3/Power Meter  Measurement=Average power  WindowLength=2000  ReferenceLoad=1  PowerUnits=dBm  SimulateUsing=Code generation
      settings: SourceProductBaseCode=DS
  Receiver Thermal Noise : commrflib2/Receiver Thermal Noise  method=Noise figure  ntemp=290  nfigure=paramRFSatLink.SatRxNoiseFigure  nfactor=2  add290KAntennaNoise=off  seed=67987
      settings: SourceProductBaseCode=CM
  Out2 : Outport
  LNA Out : Outport  Port=2
  tag scope: Cheby_Filt_Out=global, Sat_AGC_Out=global, Sat_PA_Out=global
  wires:
  Receiver Thermal Noise/1 -> LNA Out/1, Gain/1
  In1/1 -> Receiver Thermal Noise/1
  Discrete Filter/1 -> Power Meter3/1, Find Delay/2, HPA Nonlinearity/1, [Cheby_Filt_Out]
  Gain/1 -> AGC/1
  AGC/1 -> Find Delay/1, Discrete Filter/1, [Sat_AGC_Out]
  Mean3/1 -> Display Filter Output Power (dBm)/1
  Power Meter3/1 -> Mean3/1
  Power Meter1/1 -> Mean1/1
  Mean1/1 -> Display HPA Output Power (dBm)/1
  HPA Nonlinearity/1 -> Power Meter1/1, Out2/1, [Sat_PA_Out]
  Find Delay/1 -> Display/1

== system DVBS2BentPipeLinkModel/Open Intermediate Constellations ==

== system DVBS2BentPipeLinkModel/Open Eye Diagrams ==

== system DVBS2BentPipeLinkModel/Open Power Measurements ==

== system DVBS2BentPipeLinkModel/Open Received Constellation ==

== system DVBS2BentPipeLinkModel/Open Spectrum Analyzers ==

== system DVBS2BentPipeLinkModel/Open Uplink HPA AM//AM and AM//PM ==

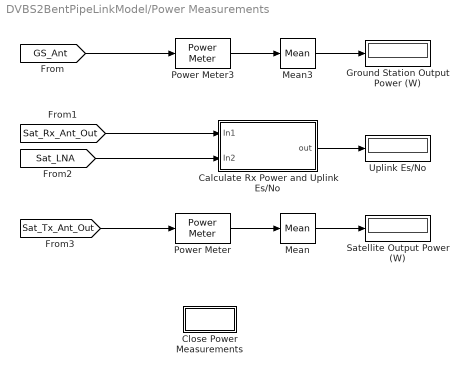
== system DVBS2BentPipeLinkModel/Power Measurements ==
  Calculate Rx Power and Uplink Es/No : Subsystem
      mask Display: disp('Calculate Rx Power\n and\nUplink Es/No')
  Close Power Measurements : Subsystem
      settings: OpenFcn=close_system([bdroot '/Power Measurements']);
      mask Display: disp('Close');
  Ground Station Output Power (W) : Display
  Mean : dspstat3/Mean  run=off  InputProcessing=Columns as channels (frame based)  reset_popup=None  directionMode=Each column  dimension=1  roiEnable=off  roiType=Rectangles  roiPortion=Entire ROI  roiOutput=Individual statistics for each ROI  roiFlag=off  roundingMode=Floor  overflowMode=off  outputDataTypeStr=Inherit: Same as accumulator  outputMin=[]  outputMax=[]  outputLastDataTypeStr=Inherit: Same as accumulator
  Mean3 : dspstat3/Mean  run=off  InputProcessing=Columns as channels (frame based)  reset_popup=None  directionMode=Each column  dimension=1  roiEnable=off  roiType=Rectangles  roiPortion=Entire ROI  roiOutput=Individual statistics for each ROI  roiFlag=off  roundingMode=Floor  overflowMode=off  outputDataTypeStr=Inherit: Same as accumulator  outputMin=[]  outputMax=[]  outputLastDataTypeStr=Inherit: Same as accumulator
  Power Meter : dspstat3/Power Meter  Measurement=Average power  WindowLength=2000  ReferenceLoad=1  PowerUnits=Watts  SimulateUsing=Code generation
      settings: SourceProductBaseCode=DS
  Power Meter3 : dspstat3/Power Meter  Measurement=Average power  WindowLength=2000  ReferenceLoad=1  PowerUnits=Watts  SimulateUsing=Code generation
      settings: SourceProductBaseCode=DS
  Satellite Output Power (W) : Display
  Uplink Es/No : Display
  wires:
  Mean3/1 -> Ground Station Output Power (W)/1
  Power Meter3/1 -> Mean3/1
  [GS_Ant] -> Power Meter3/1
  [Sat_LNA] -> Calculate Rx Power and Uplink Es/No/2(In2)
  [Sat_Rx_Ant_Out] -> Calculate Rx Power and Uplink Es/No/1(In1)
  Calculate Rx Power and Uplink Es/No/1(out) -> Uplink Es/No/1
  Power Meter/1 -> Mean/1
  [Sat_Tx_Ant_Out] -> Power Meter/1
  Mean/1 -> Satellite Output Power (W)/1

== system DVBS2BentPipeLinkModel/Power Spectra ==
  Ground Station Tx and Rx Spectra : SpectrumAnalyzer
  Matrix Concatenation : Concatenate  Mode=Multidimensional array  ConcatenateDimension=2
  Onboard Spectra : SpectrumAnalyzer  NumInputPorts=3
  wires:
  [Tx_RRC] -> Matrix Concatenation/1
  [Rx_RRC] -> Matrix Concatenation/2
  Matrix Concatenation/1 -> Ground Station Tx and Rx Spectra/1
  [Sat_AGC_Out] -> Onboard Spectra/1  "LNA Out"
  [Cheby_Filt_Out] -> Onboard Spectra/2  "Chebyshev Filter Out"
  [Sat_PA_Out] -> Onboard Spectra/3  "PA Out"

== system DVBS2BentPipeLinkModel/RF Corrections ==
  In1 : Inport
  AGC : commrfcorlib/AGC  LegacyMode=off  DetectorMethod=Rectifier  LoopMethod=Linear  UpdatePeriod=100  StepSize=0.1  AdaptationStepSize=0.01  DesiredOutputPower=1  AveragingLength=256  MaximumGain=30  MaxPowerGain=400  GainOutputPort=off  InputPowerOutputPort=off  SimulateUsing=Code generation
  DC Blocking : Subsystem
      mask Display: disp('DC Blocking')
  Doppler Correction : Subsystem
      mask Display: disp('Doppler\nCorrection')
  I/Q Imbalance Correction : Subsystem
      mask Display: disp('I/Q Imbalance\nCorrection')
  Out1 : Outport
  wires:
  Doppler Correction/1(Out1) -> Out1/1
  DC Blocking/1(Out1) -> AGC/1
  I/Q Imbalance Correction/1(Out1) -> Doppler Correction/1(In1)
  AGC/1 -> I/Q Imbalance Correction/1(In1)
  In1/1 -> DC Blocking/1(In1)

== system DVBS2BentPipeLinkModel/Received Constellation ==
  Received Constellation : ConstellationDiagram  Tag=ScatterPlot
  wires:
  [Rx_Const] -> Received Constellation/1

== system DVBS2BentPipeLinkModel/Subsystem ==

== system DVBS2BentPipeLinkModel/Subsystem1 ==

== system DVBS2BentPipeLinkModel/Subsystem2 ==

== system DVBS2BentPipeLinkModel/Subsystem3 ==

== system DVBS2BentPipeLinkModel/Subsystem4 ==

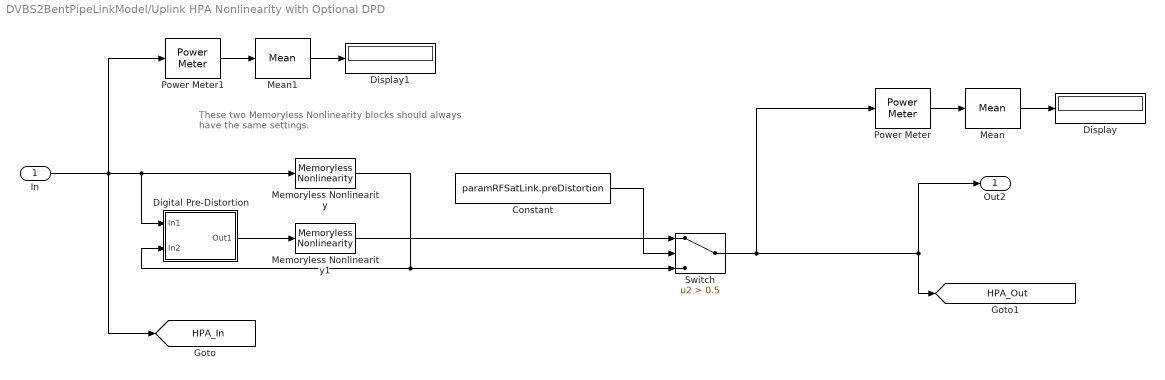
== system DVBS2BentPipeLinkModel/Uplink HPA Nonlinearity with Optional DPD ==
  note: These two Memoryless Nonlinearity blocks should always
      | have the same settings.
  In : Inport
  Constant : Constant  Value=paramRFSatLink.preDistortion  VectorParams1D=off  SampleTime="inf  % paramRFSatLink.BitPeriod"
  Digital Pre-Distortion : Subsystem
      mask Display: disp('Digital\nPredistortion')
  Display : Display
  Display1 : Display
  Mean : dspstat3/Mean  run=off  InputProcessing=Columns as channels (frame based)  reset_popup=None  directionMode=Each column  dimension=1  roiEnable=off  roiType=Rectangles  roiPortion=Entire ROI  roiOutput=Individual statistics for each ROI  roiFlag=off  roundingMode=Floor  overflowMode=off  outputDataTypeStr=Inherit: Same as accumulator  outputMin=[]  outputMax=[]  outputLastDataTypeStr=Inherit: Same as accumulator
  Mean1 : dspstat3/Mean  run=off  InputProcessing=Columns as channels (frame based)  reset_popup=None  directionMode=Each column  dimension=1  roiEnable=off  roiType=Rectangles  roiPortion=Entire ROI  roiOutput=Individual statistics for each ROI  roiFlag=off  roundingMode=Floor  overflowMode=off  outputDataTypeStr=Inherit: Same as accumulator  outputMin=[]  outputMax=[]  outputLastDataTypeStr=Inherit: Same as accumulator
  Memoryless Nonlinearity : commrflib2/Memoryless Nonlinearity  model_select=Saleh model  linGaindB=0  GindB=paramRFSatLink.GindB  iip3=30  am2pm=10  LPwrLimAMPM=10  UPwrLimAMPM=inf  amam=[2.1587 1.1517]  ampm=[4.0330 9.1040]  x=[8.1081 1.5413 6.5202 -0.0718]  y=[4.6645 2.0965 10.88 -0.003]  p=0.5  GoutdB=paramRFSatLink.GoutdB  vsat=1
      settings: SourceProductBaseCode=CM
  Memoryless Nonlinearity1 : commrflib2/Memoryless Nonlinearity  model_select=Saleh model  linGaindB=0  GindB=paramRFSatLink.GindB  iip3=30  am2pm=10  LPwrLimAMPM=10  UPwrLimAMPM=inf  amam=[2.1587 1.1517]  ampm=[4.0330 9.1040]  x=[8.1081 1.5413 6.5202 -0.0718]  y=[4.6645 2.0965 10.88 -0.003]  p=0.5  GoutdB=paramRFSatLink.GoutdB  vsat=1
      settings: SourceProductBaseCode=CM
  Power Meter : dspstat3/Power Meter  Measurement=Average power  WindowLength=2000  ReferenceLoad=1  PowerUnits=dBW  SimulateUsing=Code generation
      settings: SourceProductBaseCode=DS
  Power Meter1 : dspstat3/Power Meter  Measurement=Average power  WindowLength=2000  ReferenceLoad=1  PowerUnits=dBW  SimulateUsing=Code generation
      settings: SourceProductBaseCode=DS
  Switch : Switch  Criteria=u2 > Threshold  Threshold=0.5  ZeroCross=off
  Out2 : Outport  VectorParamsAs1DForOutWhenUnconnected=off
  tag scope: HPA_In=global, HPA_Out=global
  wires:
  Memoryless Nonlinearity/1 -> Switch/3, Digital Pre-Distortion/2(In2)
  In/1 -> Power Meter1/1, [HPA_In], Memoryless Nonlinearity/1, Digital Pre-Distortion/1(In1)
  Constant/1 -> Switch/2
  Memoryless Nonlinearity1/1 -> Switch/1
  Switch/1 -> Out2/1, [HPA_Out], Power Meter/1
  Power Meter/1 -> Mean/1
  Mean/1 -> Display/1
  Mean1/1 -> Display1/1
  Power Meter1/1 -> Mean1/1
  Digital Pre-Distortion/1(Out1) -> Memoryless Nonlinearity1/1

== system DVBS2BentPipeLinkModel/Uplink HPA AM//AM and AM//PM ==
  Input&Output of HPA : Subsystem
      mask Display: disp('Uplink HPA\nInput/Output')
  wires:
  [HPA_In] -> Input&Output of HPA/1(In1)
  [HPA_Out] -> Input&Output of HPA/2(In2)

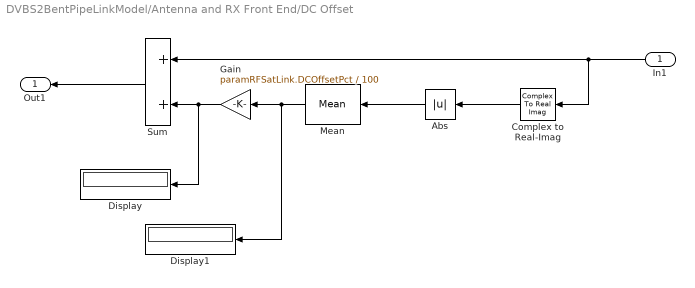
== system DVBS2BentPipeLinkModel/Antenna and RX Front End/DC Offset ==
  In1 : Inport
  Abs : Abs
  Complex to Real-Imag : ComplexToRealImag  Output=Real
  Display : Display
  Display1 : Display
  Gain : Gain  Gain=paramRFSatLink.DCOffsetPct / 100
  Mean : dspstat3/Mean  run=off  InputProcessing=Columns as channels (frame based)  reset_popup=None  directionMode=Each column  dimension=1  roiEnable=off  roiType=Rectangles  roiPortion=Entire ROI  roiOutput=Individual statistics for each ROI  roiFlag=off  roundingMode=Floor  overflowMode=off  outputDataTypeStr=Inherit: Same as accumulator  outputMin=[]  outputMax=[]  outputLastDataTypeStr=Inherit: Same as accumulator
  Sum : Sum
  Out1 : Outport
  wires:
  In1/1 -> Complex to Real-Imag/1, Sum/1
  Complex to Real-Imag/1 -> Abs/1
  Abs/1 -> Mean/1
  Mean/1 -> Display1/1, Gain/1
  Sum/1 -> Out1/1
  Gain/1 -> Display/1, Sum/2

== system DVBS2BentPipeLinkModel/Bit Source, Channel Coding, Interleaving/Buffer for Coding ==
  In1 : Inport
  Buffer : Buffer  N=paramRFSatLink.NumInfoBitsPerCodeword  OutputFrames=off
  Zero Pad : dspsigops/Pad  padAlong=Columns  dimsToPad=1  valSrc=Specify via dialog  padVal=0  spec=Output size  padNumOutRowsSpecMethod=User-specified  numOutRows=paramRFSatLink.BCHMessageLength  padNumOutColsSpecMethod=User-specified  numOutCols=1  isVarDimsMode=off  padBeginning=0  padEnd=0  outSizeMode=User-specified  outSize=1  padSigAt=End  trunc_flag=None  roundingMode=Floor  overflowMode=off  truncOrWrapMode=Truncate  wrap_flag=None
      settings: SourceProductBaseCode=DS
  Out1 : Outport  VectorParamsAs1DForOutWhenUnconnected=off
  wires:
  In1/1 -> Buffer/1
  Buffer/1 -> Zero Pad/1
  Zero Pad/1 -> Out1/1

== system DVBS2BentPipeLinkModel/Deinterleaving, Channel Decoding, Unbuffering/Unbuffer Packets ==
  In : Inport
  Buffer : Buffer  N=paramRFSatLink.NumBitsPerPacket  OutputFrames=off
  Zero Pad : dspsigops/Pad  padAlong=Columns  dimsToPad=1  valSrc=Specify via dialog  padVal=0  spec=Output size  padNumOutRowsSpecMethod=User-specified  numOutRows=paramRFSatLink.NumInfoBitsPerCodeword  padNumOutColsSpecMethod=User-specified  numOutCols=1  isVarDimsMode=off  padBeginning=0  padEnd=0  outSizeMode=User-specified  outSize=1  padSigAt=End  trunc_flag=None  roundingMode=Floor  overflowMode=off  truncOrWrapMode=Truncate  wrap_flag=None
      settings: SourceProductBaseCode=DS
  Out : Outport  VectorParamsAs1DForOutWhenUnconnected=off
  wires:
  In/1 -> Zero Pad/1
  Zero Pad/1 -> Buffer/1
  Buffer/1 -> Out/1

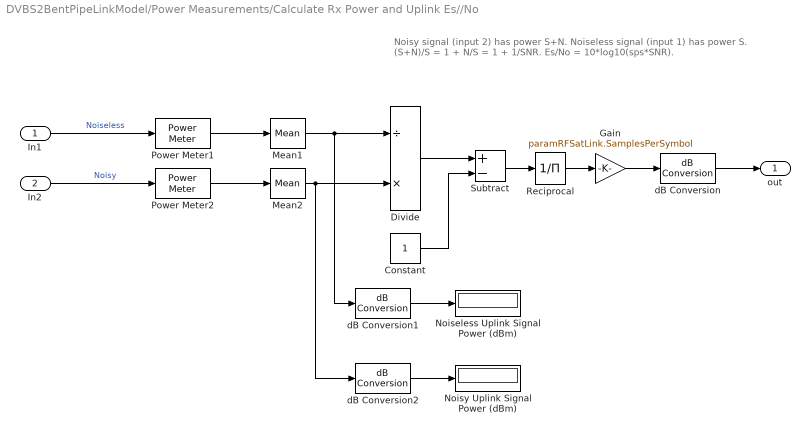
== system DVBS2BentPipeLinkModel/Power Measurements/Calculate Rx Power and Uplink Es//No ==
  note: Noisy signal (input 2) has power S+N.  Noiseless signal (input 1) has power S.
      | (S+N)/S = 1 + N/S = 1 + 1/SNR.
      | Es/No = 10*log10(sps*SNR).
  In1 : Inport
  In2 : Inport  Port=2
  Constant : Constant
  Divide : Product  Inputs=/*
  Gain : Gain  Gain=paramRFSatLink.SamplesPerSymbol
  Mean1 : dspstat3/Mean  run=off  InputProcessing=Columns as channels (frame based)  reset_popup=None  directionMode=Each column  dimension=1  roiEnable=off  roiType=Rectangles  roiPortion=Entire ROI  roiOutput=Individual statistics for each ROI  roiFlag=off  roundingMode=Floor  overflowMode=off  outputDataTypeStr=Inherit: Same as accumulator  outputMin=[]  outputMax=[]  outputLastDataTypeStr=Inherit: Same as accumulator
  Mean2 : dspstat3/Mean  run=off  InputProcessing=Columns as channels (frame based)  reset_popup=None  directionMode=Each column  dimension=1  roiEnable=off  roiType=Rectangles  roiPortion=Entire ROI  roiOutput=Individual statistics for each ROI  roiFlag=off  roundingMode=Floor  overflowMode=off  outputDataTypeStr=Inherit: Same as accumulator  outputMin=[]  outputMax=[]  outputLastDataTypeStr=Inherit: Same as accumulator
  Noiseless Uplink Signal Power (dBm) : Display
  Noisy Uplink Signal Power (dBm) : Display
  Power Meter1 : dspstat3/Power Meter  Measurement=Average power  WindowLength=2000  ReferenceLoad=1  PowerUnits=Watts  SimulateUsing=Code generation
      settings: SourceProductBaseCode=DS
  Power Meter2 : dspstat3/Power Meter  Measurement=Average power  WindowLength=2000  ReferenceLoad=1  PowerUnits=Watts  SimulateUsing=Code generation
      settings: SourceProductBaseCode=DS
  Reciprocal : Product  Inputs=/
  Subtract : Sum  Inputs=+-
  dB Conversion : dspmathops/dB Conversion  dBtype=dB  intype=Power  R=1  fuzz=off
  dB Conversion1 : dspmathops/dB Conversion  dBtype=dBm  intype=Power  R=1  fuzz=off
  dB Conversion2 : dspmathops/dB Conversion  dBtype=dBm  intype=Power  R=1  fuzz=off
  out : Outport
  wires:
  Power Meter1/1 -> Mean1/1
  Reciprocal/1 -> Gain/1
  dB Conversion1/1 -> Noiseless Uplink Signal Power (dBm)/1
  Mean2/1 -> dB Conversion2/1, Divide/2
  Divide/1 -> Subtract/1
  Mean1/1 -> dB Conversion1/1, Divide/1
  Constant/1 -> Subtract/2
  Subtract/1 -> Reciprocal/1
  Power Meter2/1 -> Mean2/1
  dB Conversion/1 -> out/1
  Gain/1 -> dB Conversion/1
  In2/1 -> Power Meter2/1  "Noisy"
  dB Conversion2/1 -> Noisy Uplink Signal Power (dBm)/1
  In1/1 -> Power Meter1/1  "Noiseless"

== system DVBS2BentPipeLinkModel/Power Measurements/Close Power Measurements ==

== system DVBS2BentPipeLinkModel/RF Corrections/DC Blocking ==
  In1 : Inport
  DC Blocker : dspsigops/DC Blocker  Algorithm=IIR  NormalizedBandwidth=0.0005  Length=8  Order=3  SimulateUsing=Code generation
      settings: SourceProductBaseCode=DS
  DC Blocker Control : Constant  Value=paramRFSatLink.DCBlock  SampleTime=Inf
  Switch : Switch  Criteria=u2 > Threshold
  Out1 : Outport  VectorParamsAs1DForOutWhenUnconnected=off
  wires:
  In1/1 -> Switch/3, DC Blocker/1
  DC Blocker Control/1 -> Switch/2
  Switch/1 -> Out1/1
  DC Blocker/1 -> Switch/1

== system DVBS2BentPipeLinkModel/RF Corrections/Doppler Correction ==
  In1 : Inport
  Carrier Synchronizer : commsync2/Carrier Synchronizer  Modulation=QPSK  ModulationPhaseOffset=Auto  CustomPhaseOffset=0  SamplesPerSymbol=1  DampingFactor=1  NormalizedLoopBandwidth=0.002  EstimatedPhaseErrorOutputPort=off  SimulateUsing=Code generation
  Doppler Correction : Constant  Value=paramRFSatLink.CarrierSync  SampleTime=Inf
  Switch : Switch  Criteria=u2 > Threshold
  Out1 : Outport  VectorParamsAs1DForOutWhenUnconnected=off
  wires:
  Doppler Correction/1 -> Switch/2
  Carrier Synchronizer/1 -> Switch/1
  Switch/1 -> Out1/1
  In1/1 -> Carrier Synchronizer/1, Switch/3

== system DVBS2BentPipeLinkModel/RF Corrections/I//Q Imbalance Correction ==
  In1 : Inport
  I/Q Imbalance Compensator : commrfcorlib/I//Q Imbalance Compensator  CoefficientSource=Estimated from input signal  InitialCoefficient=0 + 0j  StepSizeSource=Property  StepSize=0.00001  AdaptInputPort=off  CoefficientOutputPort=off  SimulateUsing=Code generation
      settings: SourceProductBaseCode=CM
  I/Q Imbalance Correction : Constant  Value=paramRFSatLink.IQComp  SampleTime=Inf
  Switch : Switch  Criteria=u2 > Threshold
  Out1 : Outport  VectorParamsAs1DForOutWhenUnconnected=off
  wires:
  I/Q Imbalance Correction/1 -> Switch/2
  I/Q Imbalance Compensator/1 -> Switch/1
  Switch/1 -> Out1/1
  In1/1 -> I/Q Imbalance Compensator/1, Switch/3

== system DVBS2BentPipeLinkModel/Uplink HPA Nonlinearity with Optional DPD/Digital Pre-Distortion ==
  In1 : Inport
  In2 : Inport  Port=2
  DPD : commrfcorlib/DPD  PolynomialType=Memory polynomial  CoefficientSource=Input port  Coefficients=complex([1 0 0 0 0; 0 0 0 0 0; 0 0 0 0 0])  SimulateUsing=Code generation
      settings: SourceProductBaseCode=CM
  DPD Coefficient Estimator : commrfcorlib/DPD Coefficient Estimator  DesiredAmplitudeGaindB=paramRFSatLink.GindB + paramRFSatLink.GoutdB  PolynomialType=Memory polynomial  Degree=1  MemoryDepth=1  Algorithm=Recursive least squares  ForgettingFactorSource=Property  ForgettingFactor=0.99  InitialCoefficientEstimate=[]  SimulateUsing=Code generation
      settings: SourceProductBaseCode=CM
  Out1 : Outport  VectorParamsAs1DForOutWhenUnconnected=off
  wires:
  In2/1 -> DPD Coefficient Estimator/2
  In1/1 -> DPD Coefficient Estimator/1, DPD/1
  DPD Coefficient Estimator/1 -> DPD/2
  DPD/1 -> Out1/1

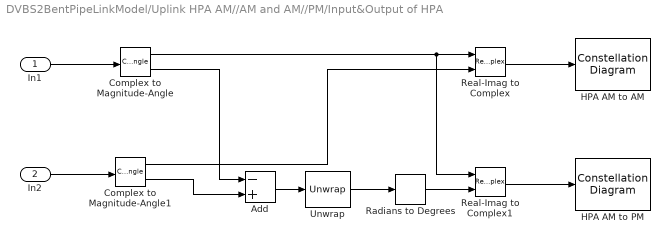
== system DVBS2BentPipeLinkModel/Uplink HPA AM//AM and AM//PM/Input&Output of HPA ==
  In1 : Inport
  In2 : Inport  Port=2
  Add : Sum  Inputs=-+
  Complex to Magnitude-Angle : ComplexToMagnitudeAngle
  Complex to Magnitude-Angle1 : ComplexToMagnitudeAngle
  HPA AM to AM : ConstellationDiagram  Tag=ScatterPlot
  HPA AM to PM : ConstellationDiagram  Tag=ScatterPlot
  Radians to Degrees : simulink_extras/Transformations/Radians to Degrees
  Real-Imag to Complex : RealImagToComplex
  Real-Imag to Complex1 : RealImagToComplex
  Unwrap : dspsigops/Unwrap  tol=pi  InputProcessing=Columns as channels (frame based)  running=on
  wires:
  Real-Imag to Complex/1 -> HPA AM to AM/1
  Complex to Magnitude-Angle1/1 -> Real-Imag to Complex/2
  Add/1 -> Unwrap/1
  In1/1 -> Complex to Magnitude-Angle/1
  In2/1 -> Complex to Magnitude-Angle1/1
  Real-Imag to Complex1/1 -> HPA AM to PM/1
  Complex to Magnitude-Angle1/2 -> Add/2
  Complex to Magnitude-Angle/1 -> Real-Imag to Complex1/1, Real-Imag to Complex/1
  Complex to Magnitude-Angle/2 -> Add/1
  Unwrap/1 -> Radians to Degrees/1
  Radians to Degrees/1 -> Real-Imag to Complex1/2
